simulink model "Q7_1"  (R2020b)
settings: Solver=VariableStepAuto  StartTime=0.0  StopTime=10  RelTol=1e-3
settings Model: Creator=Javad  LastModifiedBy=Javad

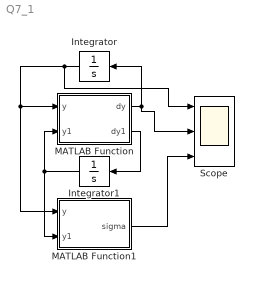
== system Q7_1 ==
  Integrator : Integrator  InitialCondition=1
  Integrator1 : Integrator
  MATLAB Function : MATLAB Function  TreatAsAtomicUnit=on
  MATLAB Function1 : MATLAB Function  TreatAsAtomicUnit=on
  Scope : Scope  NumInputPorts=3
  wires:
  MATLAB Function/2(dy1) -> Integrator1/1
  Integrator1/1 -> MATLAB Function1/2(y1), MATLAB Function/2(y1)
  MATLAB Function/1(dy) -> Integrator/1, Scope/2
  Integrator/1 -> Scope/1, MATLAB Function1/1(y), MATLAB Function/1(y)
  MATLAB Function1/1(sigma) -> Scope/3

== matlab function Q7_1/MATLAB Function ==
  data: y input; dy output; y1 input; dy1 output
function [dy,dy1] = sys(y,y1)
m=1;
b=2;
k=4;
dy=y1;
dy1=-(1/m)*(b*sign(y1)+k*y);

== matlab function Q7_1/MATLAB Function1 ==
  data: y input; sigma output; y1 input
function sigma = surface(y,y1)

sigma=y1+0.5*y;
